simulink model "durumi2_model_Vt"  (R2022a)
settings: Solver=FixedStepAuto  StartTime=0.0  StopTime=10.0  FixedStep=0.01  RelTol=1e-3  EnableMultiTasking=on
values from neighbouring files (symbols this model uses):
  x0 = [100 0 0.646770657489 0 0 0 -0.000214853328121 0.00646761624384 -1.38957920864e-06 -7.89002982394e-16 -1.35365121342e-18 -499.999868019]    [durumi2_trim_100.mat]
undefined symbols (not defined in the file or in its folder): Alpha1, Alpha2, Beta1, Beta2, cbar, CD, CL, Cl_beta, CM, CM_alpha_dot, CN_beta, Ct1, CY_beta, dCD_da_In, dCD_da_Out, dCD_de, dCD_df, dCL_da_In, dCl_da_In, dCL_da_Out, dCl_da_Out, dCL_de, dCL_df, dCl_df, dCl_dr, dCl_p, dCL_q, dCl_r, dCM_da_In, dCM_da_Out, dCM_de, dCM_df, dCM_q, dCN_dr, dCN_p, dCN_r, dCY_dr, Del_Ail_In, Del_Ail_In_f, Del_Ail_Out, Del_Ail_Out_f, Del_Ele2, Del_Flap, Del_Rud, Dp, dxcg, dzcg, g, i_th, i_throttle, Inertia, Inertia_inv, J1, L_Ail_L_In, L_Ail_L_Out, L_Ail_R_In, L_Ail_R_Out, L_Flap_L, L_Flap_R, Mass ... (+7)
libraries: simulink_extras x3, matrix_library x2, aerospace x2
settings Model: Creator=김응태  LastModifiedBy=USer
settings DataIOCC: LimitDataPoints=on  SaveFormat=Array  SignalLoggingSaveFormat=ModelDataLogs  ReturnWorkspaceOutputs=off  SignalLoggingName=sigsOut
settings DebuggingCC: SaveWithParameterizedLinksMsg=none  MergeDetectMultiDrivingBlocksExec=none  SignalResolutionControl=TryResolveAllWithWarning  MultiTaskDSMMsg=warning  MultiTaskCondExecSysMsg=none  UnconnectedInputMsg=warning  UnconnectedOutputMsg=warning  UnconnectedLineMsg=warning
settings HardwareCC: ProdBitPerPointer=32  ProdBitPerSizeT=32  ProdBitPerPtrDiffT=32  ProdLargestAtomicFloat=None  ProdIntDivRoundTo=Undefined  ProdEndianess=Unspecified  ProdWordSize=32  ProdHWDeviceType=32-bit Generic  TargetUnknown=on
settings ModelReferenceCC: PropagateSignalLabelsOutOfModel=off
settings GRTTargetCC: CombineOutputUpdateFcns=off  GRTInterface=on
settings ConfigComp: CovMetricSettings=dw  CovSaveCumulativeToWorkspaceVar=on  CovSaveSingleToWorkspaceVar=on

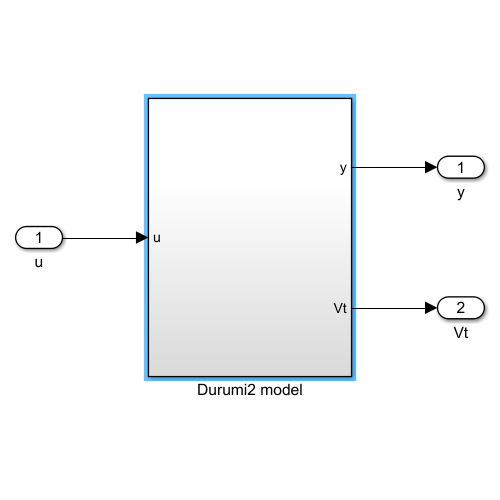
[thumbnail: Simulink's stored preview of the top-level diagram]
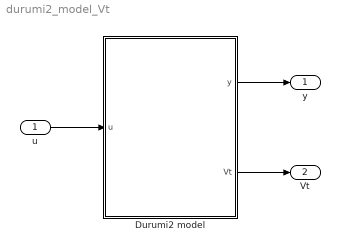
== system durumi2_model_Vt ==
  u : Inport
  Durumi2 model : Subsystem
  y : Outport
  Vt : Outport  Port=2
  wires:
  u/1 -> Durumi2 model/1(u)
  Durumi2 model/1(y) -> y/1
  Durumi2 model/2(Vt) -> Vt/1

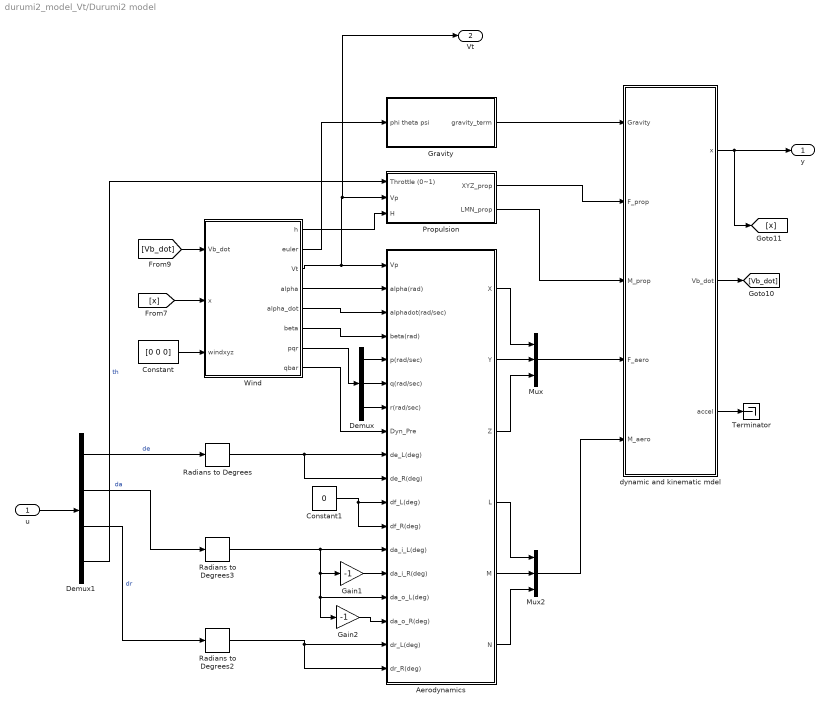
== system durumi2_model_Vt/Durumi2 model ==
  u : Inport
  "Aerodynamics " : Subsystem
  Constant : Constant  Value=[0 0 0]
  Constant1 : Constant  Value=0
  Demux : Demux  Outputs=3
      settings: DisplayOption=none
  Demux1 : Demux
  Gain1 : Gain  Gain=-1
  Gain2 : Gain  Gain=-1
  Gravity : Subsystem
  Mux : Mux  Inputs=3
  Mux2 : Mux  Inputs=3
  Propulsion : Subsystem
  Radians to Degrees : simulink_extras/Transformations/Radians to Degrees
  Radians to Degrees2 : simulink_extras/Transformations/Radians to Degrees
  Radians to Degrees3 : simulink_extras/Transformations/Radians to Degrees
  Terminator : Terminator
  Wind : Subsystem
  dynamic and kinematic mdel : Subsystem
  y : Outport
  Vt : Outport  Port=2
  wires:
  Wind/5(alpha_dot) -> "Aerodynamics "/3(alphadot(rad/sec))
  "Aerodynamics "/1(X) -> Mux/1
  Wind/8(qbar) -> "Aerodynamics "/8(Dyn_Pre)
  Wind/2(euler) -> Gravity/1(phi theta psi)
  Wind/6(beta) -> "Aerodynamics "/4(beta(rad))
  [x] -> Wind/2(x)
  [Vb_dot] -> Wind/1(Vb_dot)
  Propulsion/2(LMN_prop) -> dynamic and kinematic mdel/3(M_prop)
  Demux1/3 -> Radians to Degrees2/1  "dr"
  Propulsion/1(XYZ_prop) -> dynamic and kinematic mdel/2(F_prop)
  u/1 -> Demux1/1
  Radians to Degrees/1 -> "Aerodynamics "/10(de_R(deg)), "Aerodynamics "/9(de_L(deg))
  Constant1/1 -> "Aerodynamics "/12(df_R(deg)), "Aerodynamics "/11(df_L(deg))
  Demux1/1 -> Radians to Degrees/1  "de"
  dynamic and kinematic mdel/1(x) -> [x], y/1
  Constant/1 -> Wind/3(windxyz)
  Wind/7(pqr) -> Demux/1
  "Aerodynamics "/6(N) -> Mux2/3
  Demux/1 -> "Aerodynamics "/5(p(rad/sec))
  Wind/3(Vt) -> Vt/1, Propulsion/2(Vp), "Aerodynamics "/1(Vp)
  Demux1/2 -> Radians to Degrees3/1  "da"
  Gain2/1 -> "Aerodynamics "/16(da_o_R(deg))
  Demux/3 -> "Aerodynamics "/7(r(rad/sec))
  "Aerodynamics "/4(L) -> Mux2/1
  Mux/1 -> dynamic and kinematic mdel/4(F_aero)
  Gain1/1 -> "Aerodynamics "/14(da_i_R(deg))
  Wind/1(h) -> Propulsion/3(H)
  "Aerodynamics "/5(M) -> Mux2/2
  Gravity/1(gravity_term) -> dynamic and kinematic mdel/1(Gravity)
  dynamic and kinematic mdel/2(Vb_dot) -> [Vb_dot]
  Radians to Degrees3/1 -> "Aerodynamics "/13(da_i_L(deg)), Gain2/1, "Aerodynamics "/15(da_o_L(deg)), Gain1/1
  Demux/2 -> "Aerodynamics "/6(q(rad/sec))
  "Aerodynamics "/2(Y) -> Mux/2
  Demux1/4 -> Propulsion/1(Throttle (0~1))  "th"
  "Aerodynamics "/3(Z) -> Mux/3
  Wind/4(alpha) -> "Aerodynamics "/2(alpha(rad))
  Radians to Degrees2/1 -> "Aerodynamics "/17(dr_L(deg)), "Aerodynamics "/18(dr_R(deg))
  Mux2/1 -> dynamic and kinematic mdel/5(M_aero)
  dynamic and kinematic mdel/3(accel) -> Terminator/1

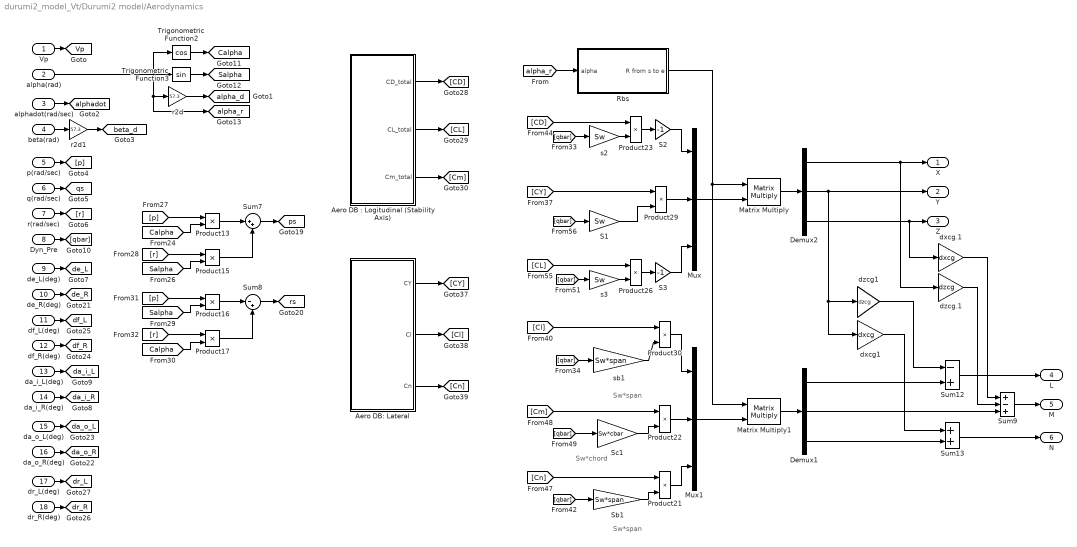
== system durumi2_model_Vt/Durumi2 model/Aerodynamics  ==
  note: Sw*span
  note: Sw*chord
  note: Sw*span
  Vp : Inport
  alpha(rad) : Inport  Port=2
  alphadot(rad/sec) : Inport  Port=3
  beta(rad) : Inport  Port=4
  p(rad/sec) : Inport  Port=5
  q(rad/sec) : Inport  Port=6
  r(rad/sec) : Inport  Port=7
  Dyn_Pre : Inport  Port=8
  de_L(deg) : Inport  Port=9
  de_R(deg) : Inport  Port=10
  df_L(deg) : Inport  Port=11
  df_R(deg) : Inport  Port=12
  da_i_L(deg) : Inport  Port=13
  da_i_R(deg) : Inport  Port=14
  da_o_L(deg) : Inport  Port=15
  da_o_R(deg) : Inport  Port=16
  dr_L(deg) : Inport  Port=17
  dr_R(deg) : Inport  Port=18
  "Aero DB : Logitudinal (Stability Axis)" : Subsystem
  Aero DB: Lateral : Subsystem
  Demux1 : Demux  Outputs=3
  Demux2 : Demux  Outputs=3
  Matrix Multiply : Product  Multiplication=Matrix(*)
  Matrix Multiply1 : Product  Multiplication=Matrix(*)
  Mux : Mux  Inputs=3
  Mux1 : Mux  Inputs=3
  Product{13,15..17,21..23,26,29..30} (10 alike) : Product  InputSameDT=on  SaturateOnIntegerOverflow=on  OutDataTypeStr=Inherit: Same as first input
  Rbs : Subsystem  AncestorBlock=|
      | aerolib6dofsys/DCM & Euler Angles (Euler)/phidot
      | thetadot
      | psidot
  S1 : Gain  Gain=Sw  SaturateOnIntegerOverflow=on  OutDataTypeStr=Inherit: Same as input  ParamDataTypeStr=Inherit: Same as input
  S2 : Gain  Gain=-1  SaturateOnIntegerOverflow=on  OutDataTypeStr=Inherit: Same as input  ParamDataTypeStr=Inherit: Same as input
  S3 : Gain  Gain=-1  SaturateOnIntegerOverflow=on  OutDataTypeStr=Inherit: Same as input  ParamDataTypeStr=Inherit: Same as input
  Sb1 : Gain  Gain=Sw*span  SaturateOnIntegerOverflow=on  OutDataTypeStr=Inherit: Same as input  ParamDataTypeStr=Inherit: Same as input
  Sc1 : Gain  Gain=Sw*cbar  SaturateOnIntegerOverflow=on  OutDataTypeStr=Inherit: Same as input  ParamDataTypeStr=Inherit: Same as input
  Sum12 : Sum  Inputs=-+  InputSameDT=on  SaturateOnIntegerOverflow=on  OutDataTypeStr=Inherit: Same as first input
  Sum13 : Sum  InputSameDT=on  SaturateOnIntegerOverflow=on  OutDataTypeStr=Inherit: Same as first input
  Sum7 : Sum  Inputs=|++  InputSameDT=on  SaturateOnIntegerOverflow=on  OutDataTypeStr=Inherit: Same as first input
  Sum8 : Sum  Inputs=|-+  InputSameDT=on  SaturateOnIntegerOverflow=on  OutDataTypeStr=Inherit: Same as first input
  Sum9 : Sum  Inputs=+-+  InputSameDT=on  SaturateOnIntegerOverflow=on  OutDataTypeStr=Inherit: Same as first input
  Trigonometric Function2 : Trigonometry  Operator=cos
  Trigonometric Function3 : Trigonometry
  dxcg.1 : Gain  Gain=dxcg  SaturateOnIntegerOverflow=on  OutDataTypeStr=Inherit: Same as input  ParamDataTypeStr=Inherit: Same as input
  dxcg1 : Gain  Gain=dxcg  SaturateOnIntegerOverflow=on  OutDataTypeStr=Inherit: Same as input  ParamDataTypeStr=Inherit: Same as input
  dzcg.1 : Gain  Gain=dzcg  SaturateOnIntegerOverflow=on  OutDataTypeStr=Inherit: Same as input  ParamDataTypeStr=Inherit: Same as input
  dzcg1 : Gain  Gain=dzcg  SaturateOnIntegerOverflow=on  OutDataTypeStr=Inherit: Same as input  ParamDataTypeStr=Inherit: Same as input
  r2d : Gain  Gain=57.3  SaturateOnIntegerOverflow=on  OutDataTypeStr=Inherit: Same as input  ParamDataTypeStr=Inherit: Same as input
  r2d1 : Gain  Gain=57.3  SaturateOnIntegerOverflow=on  OutDataTypeStr=Inherit: Same as input  ParamDataTypeStr=Inherit: Same as input
  s2 : Gain  Gain=Sw  SaturateOnIntegerOverflow=on  OutDataTypeStr=Inherit: Same as input  ParamDataTypeStr=Inherit: Same as input
  s3 : Gain  Gain=Sw  SaturateOnIntegerOverflow=on  OutDataTypeStr=Inherit: Same as input  ParamDataTypeStr=Inherit: Same as input
  sb1 : Gain  Gain=Sw*span  SaturateOnIntegerOverflow=on  OutDataTypeStr=Inherit: Same as input  ParamDataTypeStr=Inherit: Same as input
  X : Outport
  Y : Outport  Port=2
  Z : Outport  Port=3
  L : Outport  Port=4
  M : Outport  Port=5
  N : Outport  Port=6
  tag scope: Calpha=global, Salpha=global, Vp=global, alpha_d=global, alpha_r=global, alphadot=global, beta_d=global, da_i_L=global, da_i_R=global, da_o_L=global, da_o_R=global, de_L=global, de_R=global, df_L=global, df_R=global, dr_L=global, dr_R=global, ps=global, qs=global, rs=global
  wires:
  "Aero DB : Logitudinal (Stability Axis)"/3(Cm_total) -> [Cm]
  Aero DB: Lateral/3(Cn) -> [Cn]
  Aero DB: Lateral/2(Cl) -> [Cl]
  Aero DB: Lateral/1(CY) -> [CY]
  "Aero DB : Logitudinal (Stability Axis)"/2(CL_total) -> [CL]
  "Aero DB : Logitudinal (Stability Axis)"/1(CD_total) -> [CD]
  dr_R(deg)/1 -> [dr_R]
  dr_L(deg)/1 -> [dr_L]
  da_o_R(deg)/1 -> [da_o_R]
  da_o_L(deg)/1 -> [da_o_L]
  da_i_R(deg)/1 -> [da_i_R]
  da_i_L(deg)/1 -> [da_i_L]
  df_R(deg)/1 -> [df_R]
  df_L(deg)/1 -> [df_L]
  de_R(deg)/1 -> [de_R]
  Sum8/1 -> [rs]
  [r] -> Product17/1
  [p] -> Product16/1
  [Calpha] -> Product17/2
  [Salpha] -> Product16/2
  Product16/1 -> Sum8/1
  Product17/1 -> Sum8/2
  Sum7/1 -> [ps]
  [r] -> Product15/1
  [p] -> Product13/1
  [Salpha] -> Product15/2
  [Calpha] -> Product13/2
  Product13/1 -> Sum7/1
  Product15/1 -> Sum7/2
  Trigonometric Function3/1 -> [Salpha]
  Trigonometric Function2/1 -> [Calpha]
  r2d1/1 -> [beta_d]
  r2d/1 -> [alpha_d]
  Dyn_Pre/1 -> [qbar]
  alphadot(rad/sec)/1 -> [alphadot]
  beta(rad)/1 -> r2d1/1
  p(rad/sec)/1 -> [p]
  q(rad/sec)/1 -> [qs]
  r(rad/sec)/1 -> [r]
  de_L(deg)/1 -> [de_L]
  alpha(rad)/1 -> [alpha_r], r2d/1, Trigonometric Function2/1, Trigonometric Function3/1
  Vp/1 -> [Vp]
  Sb1/1 -> Product21/2
  [qbar] -> s2/1
  s3/1 -> Product26/2
  [qbar] -> S1/1
  Sc1/1 -> Product22/2
  [CD] -> Product23/1
  [CL] -> Product26/1
  s2/1 -> Product23/2
  [qbar] -> Sc1/1
  S1/1 -> Product29/2
  [qbar] -> sb1/1
  [Cl] -> Product30/1
  [CY] -> Product29/1
  [qbar] -> Sb1/1
  sb1/1 -> Product30/2
  [Cn] -> Product21/1
  [Cm] -> Product22/1
  [qbar] -> s3/1
  [alpha_r] -> Rbs/1(alpha)
  Rbs/1(R from s to e) -> Matrix Multiply/1, Matrix Multiply1/1
  Product29/1 -> Mux/2
  Product23/1 -> S2/1
  Product26/1 -> S3/1
  Product22/1 -> Mux1/2
  Product30/1 -> Mux1/1
  Product21/1 -> Mux1/3
  Mux1/1 -> Matrix Multiply1/2
  S2/1 -> Mux/1
  S3/1 -> Mux/3
  dzcg.1/1 -> Sum9/2
  dzcg1/1 -> Sum12/1
  Sum9/1 -> M/1
  Sum13/1 -> N/1
  Sum12/1 -> L/1
  Demux2/3 -> dxcg.1/1, Z/1
  Demux1/2 -> Sum9/3
  Demux1/1 -> Sum12/2
  Matrix Multiply/1 -> Demux2/1
  Matrix Multiply1/1 -> Demux1/1
  Demux2/2 -> dxcg1/1, dzcg1/1, Y/1
  dxcg.1/1 -> Sum9/1
  Demux2/1 -> X/1, dzcg.1/1
  dxcg1/1 -> Sum13/1
  Demux1/3 -> Sum13/2
  Mux/1 -> Matrix Multiply/2

== system durumi2_model_Vt/Durumi2 model/Gravity ==
  note: Gravaity
  phi theta psi : Inport
  . : Gain  Gain=g*Mass  SaturateOnIntegerOverflow=on  OutDataTypeStr=Inherit: Same as input  ParamDataTypeStr=Inherit: Same as input
  Mux : Mux  Inputs=3
  psidot2 : Fcn  Expr=cos(u[2])*cos(u[1])
  t : Fcn  Expr=-sin(u[2])
  tetadot : Fcn  Expr=cos(u[2])*sin(u[1])
  gravity_term : Outport  InitialOutput=0  VectorParamsAs1DForOutWhenUnconnected=off
  wires:
  t/1 -> Mux/1
  psidot2/1 -> Mux/3
  tetadot/1 -> Mux/2
  Mux/1 -> ./1
  phi theta psi/1 -> tetadot/1, t/1, psidot2/1
  ./1 -> gravity_term/1

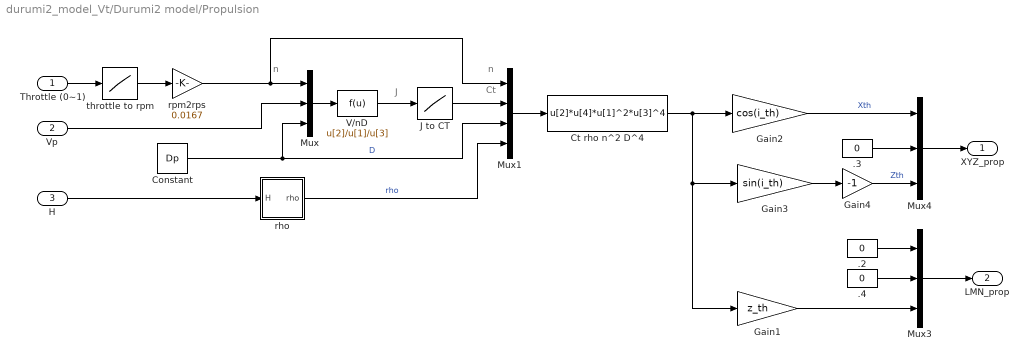
== system durumi2_model_Vt/Durumi2 model/Propulsion ==
  note: Ct
  note: n
  note: J
  note: n
  Throttle (0~1) : Inport
  Vp : Inport  Port=2
  H : Inport  Port=3
  .2 : Constant  Value=0  VectorParams1D=off
  .3 : Constant  Value=0  VectorParams1D=off
  .4 : Constant  Value=0  VectorParams1D=off
  Constant : Constant  Value=Dp
  Ct rho n^2 D^4 : Fcn  Expr=u[2]*u[4]*u[1]^2*u[3]^4
  Gain1 : Gain  Gain=z_th  SaturateOnIntegerOverflow=on  OutDataTypeStr=Inherit: Same as input  ParamDataTypeStr=Inherit: Same as input
  Gain2 : Gain  Gain=cos(i_th)  SaturateOnIntegerOverflow=on  OutDataTypeStr=Inherit: Same as input  ParamDataTypeStr=Inherit: Same as input
  Gain3 : Gain  Gain=sin(i_th)  SaturateOnIntegerOverflow=on  OutDataTypeStr=Inherit: Same as input  ParamDataTypeStr=Inherit: Same as input
  Gain4 : Gain  Gain=-1  SaturateOnIntegerOverflow=on  OutDataTypeStr=Inherit: Same as input  ParamDataTypeStr=Inherit: Same as input
  J to CT : Lookup  InputValues=J1  Table=Ct1
  Mux : Mux  Inputs=3
  Mux1 : Mux
  Mux3 : Mux  Inputs=3
  Mux4 : Mux  Inputs=3
  V/nD : Fcn  Expr=u[2]/u[1]/u[3]
  rho : Subsystem
  rpm2rps : Gain  Gain=0.0167  SaturateOnIntegerOverflow=on  OutDataTypeStr=Inherit: Same as input  ParamDataTypeStr=Inherit: Same as input
  throttle to rpm : Lookup  InputValues=i_throttle  Table=o_rpm
  XYZ_prop : Outport  VectorParamsAs1DForOutWhenUnconnected=off
  LMN_prop : Outport  Port=2  VectorParamsAs1DForOutWhenUnconnected=off
  wires:
  .3/1 -> Mux4/2
  Mux4/1 -> XYZ_prop/1
  Ct rho n^2 D^4/1 -> Gain2/1, Gain3/1, Gain1/1
  Gain1/1 -> Mux3/3
  Gain3/1 -> Gain4/1
  Mux3/1 -> LMN_prop/1
  .4/1 -> Mux3/2
  .2/1 -> Mux3/1
  Gain2/1 -> Mux4/1  "Xth"
  Gain4/1 -> Mux4/3  "Zth"
  rho/1(rho) -> Mux1/4  "rho"
  J to CT/1 -> Mux1/2
  Vp/1 -> Mux/2
  Mux/1 -> V/nD/1
  Mux1/1 -> Ct rho n^2 D^4/1
  V/nD/1 -> J to CT/1
  Constant/1 -> Mux1/3, Mux/3  "D"
  H/1 -> rho/1(H)
  Throttle (0~1)/1 -> throttle to rpm/1
  throttle to rpm/1 -> rpm2rps/1
  rpm2rps/1 -> Mux/1, Mux1/1

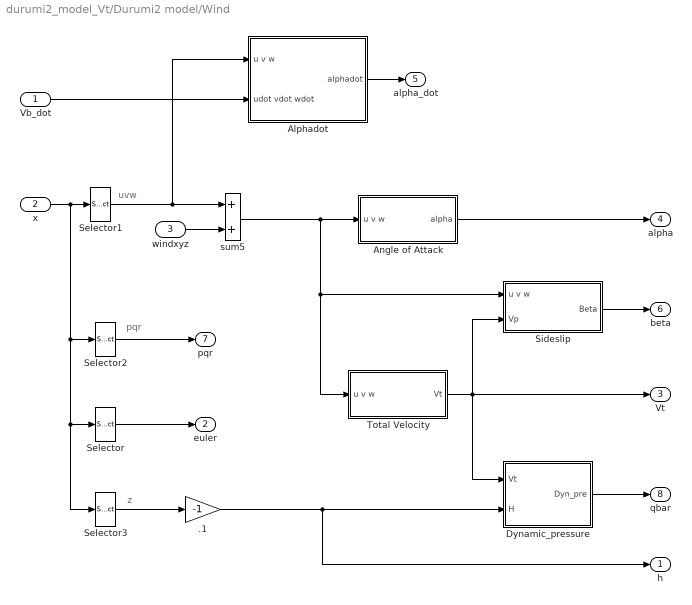
== system durumi2_model_Vt/Durumi2 model/Wind ==
  note: uvw
  note: pqr
  note: z
  Vb_dot : Inport
  x : Inport  Port=2
  windxyz : Inport  Port=3
  .1 : Gain  Gain=-1  OutDataTypeStr=Inherit: Same as input  ParamDataTypeStr=Inherit: Same as input
  Alphadot : Subsystem
  Angle of Attack : Subsystem
  Dynamic_pressure : Subsystem
  Selector : Selector  InputPortWidth=12  IndexOptions=Index vector (dialog)  Indices=[7 8 9]  OutputSizes=1
  Selector1 : Selector  InputPortWidth=12  IndexOptions=Index vector (dialog)  Indices=[1 2 3]  OutputSizes=1
  Selector2 : Selector  InputPortWidth=12  IndexOptions=Index vector (dialog)  Indices=[4 5 6]  OutputSizes=1
  Selector3 : Selector  InputPortWidth=12  IndexOptions=Index vector (dialog)  Indices=12  OutputSizes=1
  Sideslip : Subsystem
  Total Velocity : Subsystem
  sum5 : Sum  InputSameDT=on  SaturateOnIntegerOverflow=on  OutDataTypeStr=Inherit: Same as first input
  h : Outport  VectorParamsAs1DForOutWhenUnconnected=off
  euler : Outport  Port=2  VectorParamsAs1DForOutWhenUnconnected=off
  Vt : Outport  Port=3  VectorParamsAs1DForOutWhenUnconnected=off
  alpha : Outport  Port=4  VectorParamsAs1DForOutWhenUnconnected=off
  alpha_dot : Outport  Port=5  VectorParamsAs1DForOutWhenUnconnected=off
  beta : Outport  Port=6  VectorParamsAs1DForOutWhenUnconnected=off
  pqr : Outport  Port=7  VectorParamsAs1DForOutWhenUnconnected=off
  qbar : Outport  Port=8  VectorParamsAs1DForOutWhenUnconnected=off
  wires:
  x/1 -> Selector/1, Selector3/1, Selector2/1, Selector1/1
  Selector3/1 -> .1/1
  Angle of Attack/1(alpha) -> alpha/1
  Sideslip/1(Beta) -> beta/1
  windxyz/1 -> sum5/2
  Selector2/1 -> pqr/1
  sum5/1 -> Sideslip/1(u v w), Total Velocity/1(u v w), Angle of Attack/1(u v w)
  .1/1 -> Dynamic_pressure/2(H), h/1
  Total Velocity/1(Vt) -> Dynamic_pressure/1(Vt), Sideslip/2(Vp), Vt/1
  Dynamic_pressure/1(Dyn_pre) -> qbar/1
  Selector1/1 -> Alphadot/1(u v w), sum5/1
  Alphadot/1(alphadot) -> alpha_dot/1
  Vb_dot/1 -> Alphadot/2(udot vdot wdot)
  Selector/1 -> euler/1

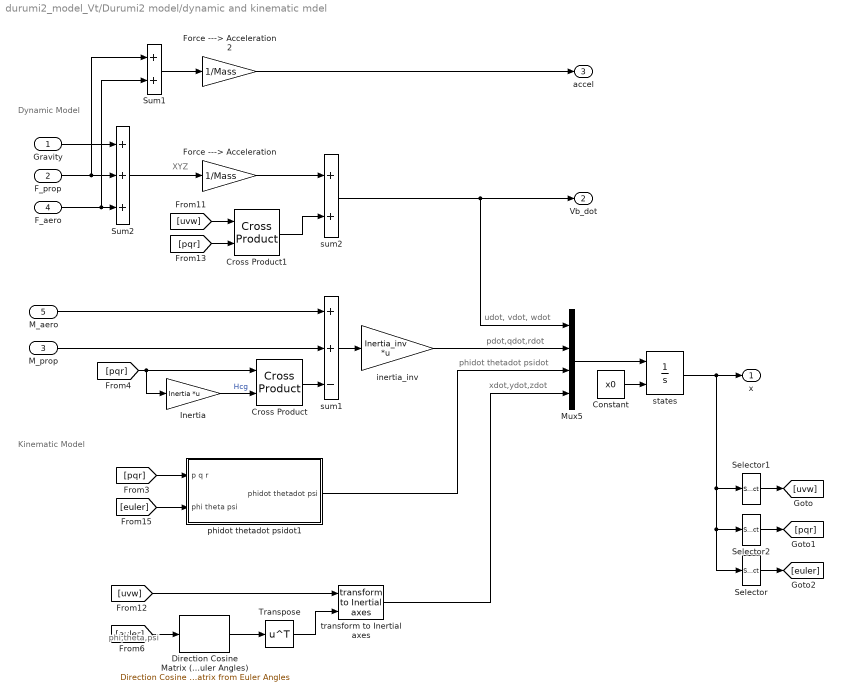
== system durumi2_model_Vt/Durumi2 model/dynamic and kinematic mdel ==
  note: Dynamic Model
  note: XYZ
  note: xdot,ydot,zdot
  note: phidot thetadot psidot
  note: pdot,qdot,rdot
  note: udot, vdot, wdot
  note: phi,theta,psi
  note: Kinematic Model
  Gravity : Inport
  F_prop : Inport  Port=2
  M_prop : Inport  Port=3
  F_aero : Inport  Port=4
  M_aero : Inport  Port=5
  Constant : Constant  Value=x0
  Cross Product : matrix_library/Cross Product
      settings: SourceProductBaseCode=SL
  Cross Product1 : matrix_library/Cross Product
      settings: SourceProductBaseCode=SL
  Direction Cosine Matrix (Euler Angles) : aerospace/Axes Transformations/Direction Cosine Matrix from Euler Angles
      settings: SourceProductBaseCode=SL
  Force ---> Acceleration : Gain  Gain=1/Mass  SaturateOnIntegerOverflow=on  OutDataTypeStr=Inherit: Same as input  ParamDataTypeStr=Inherit: Same as input
  Force ---> Acceleration2 : Gain  Gain=1/Mass  SaturateOnIntegerOverflow=on  OutDataTypeStr=Inherit: Same as input  ParamDataTypeStr=Inherit: Same as input
  Inertia : Gain  Gain=Inertia  Multiplication=Matrix(K*u)
  Mux5 : Mux
  Selector : Selector  InputPortWidth=12  IndexOptions=Index vector (dialog)  Indices=[7 8 9]  OutputSizes=1
  Selector1 : Selector  InputPortWidth=12  IndexOptions=Index vector (dialog)  Indices=[1 2 3]  OutputSizes=1
  Selector2 : Selector  InputPortWidth=12  IndexOptions=Index vector (dialog)  Indices=[4 5 6]  OutputSizes=1
  Sum1 : Sum  InputSameDT=on  SaturateOnIntegerOverflow=on  OutDataTypeStr=Inherit: Same as first input
  Sum2 : Sum  Inputs=+++  InputSameDT=on  SaturateOnIntegerOverflow=on  OutDataTypeStr=Inherit: Same as first input
  Transpose : Math  Operator=transpose  SignedPower=on
  inertia_inv : Gain  Gain=Inertia_inv  Multiplication=Matrix(K*u)
  phidot thetadot psidot1 : Subsystem  AncestorBlock=|
      | aerolib6dofsys/DCM & Euler Angles (Euler)/phidot
      | thetadot
      | psidot
  states : Integrator  InitialConditionSource=external  InitialCondition=x0
  sum1 : Sum  Inputs=++-  InputSameDT=on  SaturateOnIntegerOverflow=on  OutDataTypeStr=Inherit: Same as first input
  sum2 : Sum  InputSameDT=on  SaturateOnIntegerOverflow=on  OutDataTypeStr=Inherit: Same as first input
  "transform to Inertial axes " : aerospace/6DoF/Euler Angles/transform to Inertial axes   SystemSampleTime=-1  VariantActivationTime=update diagram  Latency=0  AutoFrameSizeCalculation=off
      settings: SourceProductBaseCode=SL
  x : Outport  VectorParamsAs1DForOutWhenUnconnected=off
  Vb_dot : Outport  Port=2  VectorParamsAs1DForOutWhenUnconnected=off
  accel : Outport  Port=3  VectorParamsAs1DForOutWhenUnconnected=off
  wires:
  Selector/1 -> [euler]
  Constant/1 -> states/2
  Selector1/1 -> [uvw]
  states/1 -> x/1, Selector2/1, Selector/1, Selector1/1
  Selector2/1 -> [pqr]
  [euler] -> Direction Cosine Matrix (Euler Angles)/1
  [pqr] -> phidot thetadot psidot1/1(p q r)
  "transform to Inertial axes "/1 -> Mux5/4
  [euler] -> phidot thetadot psidot1/2(phi theta psi)
  [pqr] -> Cross Product1/2
  [uvw] -> "transform to Inertial axes "/1
  [uvw] -> Cross Product1/1
  [pqr] -> Cross Product/1, Inertia/1
  Mux5/1 -> states/1
  inertia_inv/1 -> Mux5/2
  Transpose/1 -> "transform to Inertial axes "/2
  sum2/1 -> Vb_dot/1, Mux5/1
  Direction Cosine Matrix (Euler Angles)/1 -> Transpose/1
  phidot thetadot psidot1/1(phidot thetadot psi) -> Mux5/3
  Inertia/1 -> Cross Product/2  "Hcg"
  sum1/1 -> inertia_inv/1
  Cross Product1/1 -> sum2/2
  Force ---> Acceleration/1 -> sum2/1
  Sum2/1 -> Force ---> Acceleration/1
  F_prop/1 -> Sum1/1, Sum2/2
  F_aero/1 -> Sum1/2, Sum2/3
  M_aero/1 -> sum1/1
  Cross Product/1 -> sum1/3
  M_prop/1 -> sum1/2
  Sum1/1 -> Force ---> Acceleration2/1
  Gravity/1 -> Sum2/1
  Force ---> Acceleration2/1 -> accel/1

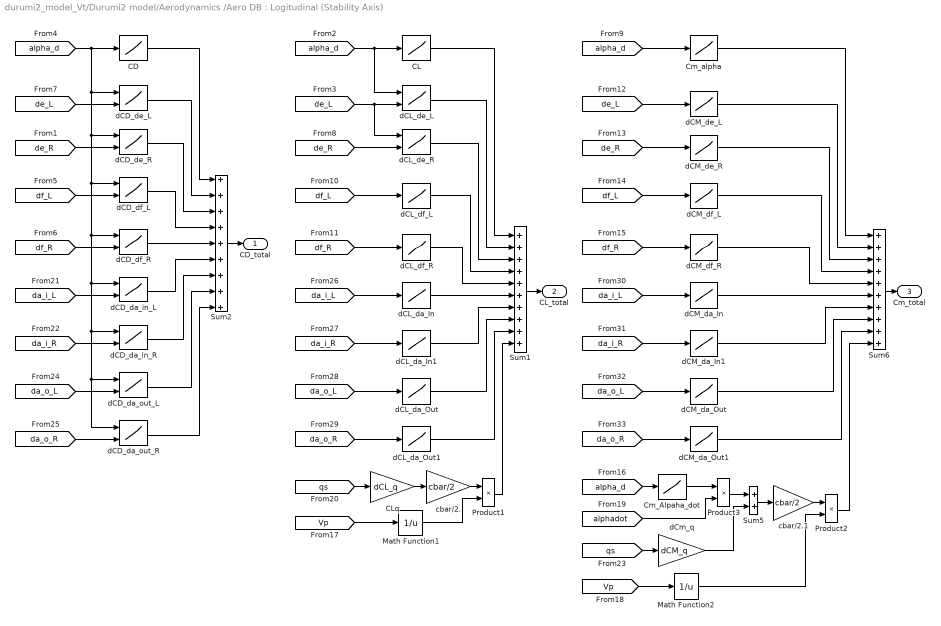
== system durumi2_model_Vt/Durumi2 model/Aerodynamics /Aero DB : Logitudinal (Stability Axis) ==
  CD : Lookup  InputValues=Alpha1  Table=CD
  CL : Lookup  InputValues=Alpha2  Table=CL
  CLq : Gain  Gain=dCL_q  SaturateOnIntegerOverflow=on  OutDataTypeStr=Inherit: Same as input  ParamDataTypeStr=Inherit: Same as input
  Cm_Alpaha_dot : Lookup  InputValues=Alpha2  Table=CM_alpha_dot
  Cm_alpha : Lookup  InputValues=Alpha2  Table=CM
  Math Function1 : Math  Operator=reciprocal  SignedPower=on
  Math Function2 : Math  Operator=reciprocal  SignedPower=on
  Product1 : Product  InputSameDT=on  SaturateOnIntegerOverflow=on  OutDataTypeStr=Inherit: Same as first input
  Product2 : Product  InputSameDT=on  SaturateOnIntegerOverflow=on  OutDataTypeStr=Inherit: Same as first input
  Product3 : Product  InputSameDT=on  SaturateOnIntegerOverflow=on  OutDataTypeStr=Inherit: Same as first input
  Sum1 : Sum  Inputs=++++++++++  InputSameDT=on  SaturateOnIntegerOverflow=on  OutDataTypeStr=Inherit: Same as first input
  Sum2 : Sum  Inputs=+++++++++  InputSameDT=on  SaturateOnIntegerOverflow=on  OutDataTypeStr=Inherit: Same as first input
  Sum5 : Sum  InputSameDT=on  SaturateOnIntegerOverflow=on  OutDataTypeStr=Inherit: Same as first input
  Sum6 : Sum  Inputs=++++++++++  InputSameDT=on  SaturateOnIntegerOverflow=on  OutDataTypeStr=Inherit: Same as first input
  cbar/2. : Gain  Gain=cbar/2  SaturateOnIntegerOverflow=on  OutDataTypeStr=Inherit: Same as input  ParamDataTypeStr=Inherit: Same as input
  cbar/2.1 : Gain  Gain=cbar/2  SaturateOnIntegerOverflow=on  OutDataTypeStr=Inherit: Same as input  ParamDataTypeStr=Inherit: Same as input
  dCD_da_in_L : Lookup2D  RowIndex=Alpha2  ColumnIndex=Del_Ail_In_f  Table=dCD_da_In  InputSameDT=off
  dCD_da_in_R : Lookup2D  RowIndex=Alpha2  ColumnIndex=Del_Ail_In_f  Table=dCD_da_In  InputSameDT=off
  dCD_da_out_L : Lookup2D  RowIndex=Alpha2  ColumnIndex=Del_Ail_Out_f  Table=dCD_da_Out  InputSameDT=off
  dCD_da_out_R : Lookup2D  RowIndex=Alpha2  ColumnIndex=Del_Ail_Out_f  Table=dCD_da_Out  InputSameDT=off
  dCD_de_L : Lookup2D  RowIndex=Alpha1  ColumnIndex=Del_Ele1  Table=dCD_de  InputSameDT=off
  dCD_de_R : Lookup2D  RowIndex=Alpha1  ColumnIndex=Del_Ele1  Table=dCD_de  InputSameDT=off
  dCD_df_L : Lookup2D  RowIndex=Alpha2  ColumnIndex=Del_Flap  Table=dCD_df  InputSameDT=off
  dCD_df_R : Lookup2D  RowIndex=Alpha2  ColumnIndex=Del_Flap  Table=dCD_df  InputSameDT=off
  dCL_da_In : Lookup  InputValues=Del_Ail_In_f  Table=dCL_da_In
  dCL_da_In1 : Lookup  InputValues=Del_Ail_In_f  Table=dCL_da_In
  dCL_da_Out : Lookup  InputValues=Del_Ail_Out_f  Table=dCL_da_Out
  dCL_da_Out1 : Lookup  InputValues=Del_Ail_Out_f  Table=dCL_da_Out
  dCL_de_L : Lookup2D  RowIndex=Alpha1  ColumnIndex=Del_Ele1  Table=dCL_de  InputSameDT=off
  dCL_de_R : Lookup2D  RowIndex=Alpha1  ColumnIndex=Del_Ele1  Table=dCL_de  InputSameDT=off
  dCL_df_L : Lookup  InputValues=Del_Flap  Table=dCL_df
  dCL_df_R : Lookup  InputValues=Del_Flap  Table=dCL_df
  dCM_da_In : Lookup  InputValues=Del_Ail_In_f  Table=dCM_da_In
  dCM_da_In1 : Lookup  InputValues=Del_Ail_In_f  Table=dCM_da_In
  dCM_da_Out : Lookup  InputValues=Del_Ail_Out_f  Table=dCM_da_Out
  dCM_da_Out1 : Lookup  InputValues=Del_Ail_Out_f  Table=dCM_da_Out
  dCM_de_L : Lookup  InputValues=Del_Ele2  Table=dCM_de
  dCM_de_R : Lookup  InputValues=Del_Ele2  Table=dCM_de
  dCM_df_L : Lookup  InputValues=Del_Flap  Table=dCM_df
  dCM_df_R : Lookup  InputValues=Del_Flap  Table=dCM_df
  dCm_q : Gain  Gain=dCM_q  SaturateOnIntegerOverflow=on  OutDataTypeStr=Inherit: Same as input  ParamDataTypeStr=Inherit: Same as input
  CD_total : Outport
  CL_total : Outport  Port=2
  Cm_total : Outport  Port=3
  wires:
  dCM_da_Out/1 -> Sum6/8
  dCM_da_In1/1 -> Sum6/7
  dCM_da_In/1 -> Sum6/6
  dCM_da_Out1/1 -> Sum6/9
  Product2/1 -> Sum6/10
  [da_o_R] -> dCM_da_Out1/1
  [da_o_L] -> dCM_da_Out/1
  [da_i_R] -> dCM_da_In1/1
  [da_i_L] -> dCM_da_In/1
  dCL_da_In1/1 -> Sum1/7
  dCL_da_Out/1 -> Sum1/8
  Product1/1 -> Sum1/10
  dCL_da_Out1/1 -> Sum1/9
  dCL_da_In/1 -> Sum1/6
  [da_o_R] -> dCL_da_Out1/1
  [da_o_L] -> dCL_da_Out/1
  [da_i_R] -> dCL_da_In1/1
  [da_i_L] -> dCL_da_In/1
  dCD_da_out_R/1 -> Sum2/9
  dCD_da_out_L/1 -> Sum2/8
  dCD_da_in_R/1 -> Sum2/7
  dCD_da_in_L/1 -> Sum2/6
  [da_o_R] -> dCD_da_out_R/2
  [da_o_L] -> dCD_da_out_L/2
  [da_i_R] -> dCD_da_in_R/2
  [da_i_L] -> dCD_da_in_L/2
  dCm_q/1 -> Sum5/2
  [alphadot] -> Product3/2
  Product3/1 -> Sum5/1
  Cm_Alpaha_dot/1 -> Product3/1
  Math Function1/1 -> Product1/2
  cbar/2./1 -> Product1/1
  CLq/1 -> cbar/2./1
  [Vp] -> Math Function1/1
  [qs] -> CLq/1
  dCM_de_L/1 -> Sum6/2
  Cm_alpha/1 -> Sum6/1
  dCM_df_R/1 -> Sum6/5
  dCM_de_R/1 -> Sum6/3
  dCM_df_L/1 -> Sum6/4
  Math Function2/1 -> Product2/2
  cbar/2.1/1 -> Product2/1
  Sum5/1 -> cbar/2.1/1
  [Vp] -> Math Function2/1
  [qs] -> dCm_q/1
  [alpha_d] -> Cm_Alpaha_dot/1
  [df_R] -> dCM_df_R/1
  [df_L] -> dCM_df_L/1
  [de_R] -> dCM_de_R/1
  [de_L] -> dCM_de_L/1
  [alpha_d] -> Cm_alpha/1
  Sum1/1 -> CL_total/1
  dCL_df_R/1 -> Sum1/5
  CL/1 -> Sum1/1
  dCL_df_L/1 -> Sum1/4
  dCL_de_L/1 -> Sum1/2
  dCL_de_R/1 -> Sum1/3
  [df_R] -> dCL_df_R/1
  [df_L] -> dCL_df_L/1
  [de_R] -> dCL_de_R/2
  [alpha_d] -> dCL_de_L/1, CL/1
  [df_R] -> dCD_df_R/2
  [df_L] -> dCD_df_L/2
  dCD_df_R/1 -> Sum2/5
  [de_R] -> dCD_de_R/2
  [de_L] -> dCD_de_L/2
  Sum6/1 -> Cm_total/1
  dCD_df_L/1 -> Sum2/4
  dCD_de_R/1 -> Sum2/3
  Sum2/1 -> CD_total/1
  dCD_de_L/1 -> Sum2/2
  CD/1 -> Sum2/1
  [alpha_d] -> dCD_da_out_R/1, dCD_da_out_L/1, dCD_da_in_R/1, dCD_da_in_L/1, dCD_df_R/1, dCD_df_L/1, dCD_de_R/1, dCD_de_L/1, CD/1
  [de_L] -> dCL_de_R/1, dCL_de_L/2

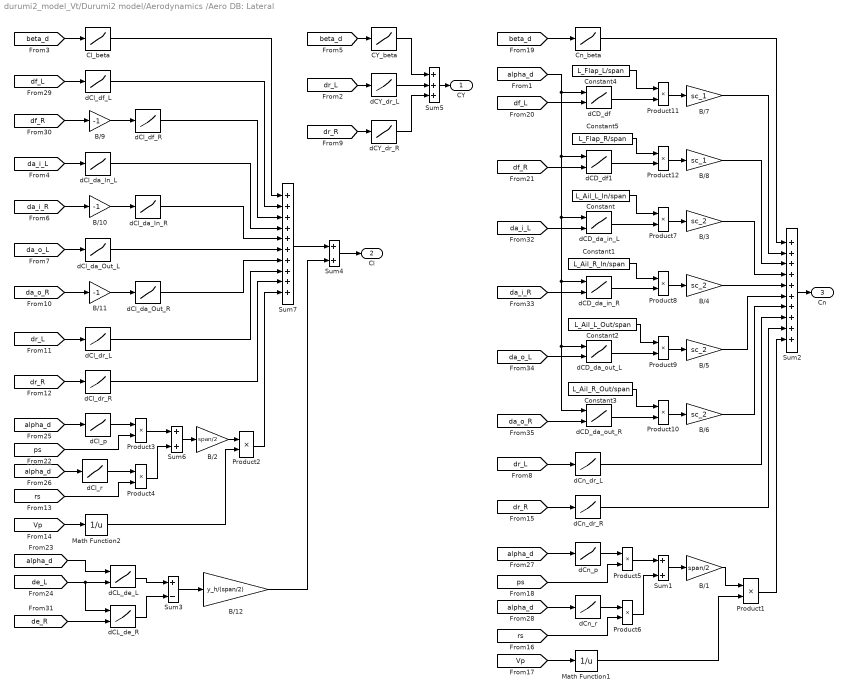
== system durumi2_model_Vt/Durumi2 model/Aerodynamics /Aero DB: Lateral ==
  B/1 : Gain  Gain=span/2  SaturateOnIntegerOverflow=on  OutDataTypeStr=Inherit: Same as input  ParamDataTypeStr=Inherit: Same as input
  B/10 : Gain  Gain=-1  SaturateOnIntegerOverflow=on  OutDataTypeStr=Inherit: Same as input  ParamDataTypeStr=Inherit: Same as input
  B/11 : Gain  Gain=-1  SaturateOnIntegerOverflow=on  OutDataTypeStr=Inherit: Same as input  ParamDataTypeStr=Inherit: Same as input
  B/12 : Gain  Gain=y_h/(span/2)  SaturateOnIntegerOverflow=on  OutDataTypeStr=Inherit: Same as input  ParamDataTypeStr=Inherit: Same as input
  B/2 : Gain  Gain=span/2  SaturateOnIntegerOverflow=on  OutDataTypeStr=Inherit: Same as input  ParamDataTypeStr=Inherit: Same as input
  B/{3..6} (4 alike) : Gain  Gain=sc_2  SaturateOnIntegerOverflow=on  OutDataTypeStr=Inherit: Same as input  ParamDataTypeStr=Inherit: Same as input
  B/7 : Gain  Gain=sc_1  SaturateOnIntegerOverflow=on  OutDataTypeStr=Inherit: Same as input  ParamDataTypeStr=Inherit: Same as input
  B/8 : Gain  Gain=sc_1  SaturateOnIntegerOverflow=on  OutDataTypeStr=Inherit: Same as input  ParamDataTypeStr=Inherit: Same as input
  B/9 : Gain  Gain=-1  SaturateOnIntegerOverflow=on  OutDataTypeStr=Inherit: Same as input  ParamDataTypeStr=Inherit: Same as input
  CY_beta : Lookup  InputValues=Beta1  Table=CY_beta
  Cl_beta : Lookup  InputValues=Beta2  Table=Cl_beta
  Cn_beta : Lookup  InputValues=Beta1  Table=CN_beta
  Constant : Constant  Value=L_Ail_L_In/span
  Constant1 : Constant  Value=L_Ail_R_In/span
  Constant2 : Constant  Value=L_Ail_L_Out/span
  Constant3 : Constant  Value=L_Ail_R_Out/span
  Constant4 : Constant  Value=L_Flap_L/span
  Constant5 : Constant  Value=L_Flap_R/span
  Math Function1 : Math  Operator=reciprocal  SignedPower=on
  Math Function2 : Math  Operator=reciprocal  SignedPower=on
  Product{1..12} (12 alike) : Product  InputSameDT=on  SaturateOnIntegerOverflow=on  OutDataTypeStr=Inherit: Same as first input
  Sum1 : Sum  InputSameDT=on  SaturateOnIntegerOverflow=on  OutDataTypeStr=Inherit: Same as first input
  Sum2 : Sum  Inputs=++++++++++  InputSameDT=on  SaturateOnIntegerOverflow=on  OutDataTypeStr=Inherit: Same as first input
  Sum3 : Sum  Inputs=+-  InputSameDT=on  SaturateOnIntegerOverflow=on  OutDataTypeStr=Inherit: Same as first input
  Sum4 : Sum  InputSameDT=on  SaturateOnIntegerOverflow=on  OutDataTypeStr=Inherit: Same as first input
  Sum5 : Sum  Inputs=+++  InputSameDT=on  SaturateOnIntegerOverflow=on  OutDataTypeStr=Inherit: Same as first input
  Sum6 : Sum  InputSameDT=on  SaturateOnIntegerOverflow=on  OutDataTypeStr=Inherit: Same as first input
  Sum7 : Sum  Inputs=++++++++++  InputSameDT=on  SaturateOnIntegerOverflow=on  OutDataTypeStr=Inherit: Same as first input
  dCD_da_in_L : Lookup2D  RowIndex=Alpha2  ColumnIndex=Del_Ail_In_f  Table=dCD_da_In  InputSameDT=off
  dCD_da_in_R : Lookup2D  RowIndex=Alpha2  ColumnIndex=Del_Ail_In_f  Table=dCD_da_In  InputSameDT=off
  dCD_da_out_L : Lookup2D  RowIndex=Alpha2  ColumnIndex=Del_Ail_Out_f  Table=dCD_da_Out  InputSameDT=off
  dCD_da_out_R : Lookup2D  RowIndex=Alpha2  ColumnIndex=Del_Ail_Out_f  Table=dCD_da_Out  InputSameDT=off
  dCD_df : Lookup2D  RowIndex=Alpha2  ColumnIndex=Del_Flap  Table=dCD_df  InputSameDT=off
  dCD_df1 : Lookup2D  RowIndex=Alpha2  ColumnIndex=Del_Flap  Table=dCD_df  InputSameDT=off
  dCL_de_L : Lookup2D  RowIndex=Alpha1  ColumnIndex=Del_Ele1  Table=dCL_de  InputSameDT=off
  dCL_de_R : Lookup2D  RowIndex=Alpha1  ColumnIndex=Del_Ele1  Table=dCL_de  InputSameDT=off
  dCY_dr_L : Lookup  InputValues=Del_Rud  Table=dCY_dr
  dCY_dr_R : Lookup  InputValues=Del_Rud  Table=dCY_dr
  dCl_da_In_L : Lookup  InputValues=Del_Ail_In  Table=dCl_da_In
  dCl_da_In_R : Lookup  InputValues=Del_Ail_In  Table=dCl_da_In
  dCl_da_Out_L : Lookup  InputValues=Del_Ail_Out  Table=dCl_da_Out
  dCl_da_Out_R : Lookup  InputValues=Del_Ail_Out  Table=dCl_da_Out
  dCl_df_L : Lookup  InputValues=Del_Flap  Table=dCl_df
  dCl_df_R : Lookup  InputValues=Del_Flap  Table=dCl_df
  dCl_dr_L : Lookup  InputValues=Del_Rud  Table=dCl_dr
  dCl_dr_R : Lookup  InputValues=Del_Rud  Table=dCl_dr
  dCl_p : Lookup  InputValues=Alpha2  Table=dCl_p
  dCl_r : Lookup  InputValues=Alpha2  Table=dCl_r
  dCn_dr_L : Lookup  InputValues=Del_Rud  Table=dCN_dr
  dCn_dr_R : Lookup  InputValues=Del_Rud  Table=dCN_dr
  dCn_p : Lookup  InputValues=Alpha2  Table=dCN_p
  dCn_r : Lookup  InputValues=Alpha2  Table=dCN_r
  CY : Outport
  Cl : Outport  Port=2
  Cn : Outport  Port=3
  wires:
  B/12/1 -> Sum4/2
  Sum3/1 -> B/12/1
  Sum4/1 -> Cl/1
  Sum7/1 -> Sum4/1
  dCL_de_R/1 -> Sum3/2
  dCL_de_L/1 -> Sum3/1
  [de_R] -> dCL_de_R/2
  [alpha_d] -> dCL_de_L/1
  [de_L] -> dCL_de_R/1, dCL_de_L/2
  B/11/1 -> dCl_da_Out_R/1
  B/10/1 -> dCl_da_In_R/1
  B/9/1 -> dCl_df_R/1
  Product1/1 -> Sum2/10
  dCn_dr_R/1 -> Sum2/9
  dCn_dr_L/1 -> Sum2/8
  B/6/1 -> Sum2/7
  B/5/1 -> Sum2/6
  B/4/1 -> Sum2/5
  B/3/1 -> Sum2/4
  B/8/1 -> Sum2/3
  B/7/1 -> Sum2/2
  Product12/1 -> B/8/1
  Product11/1 -> B/7/1
  Constant5/1 -> Product12/1
  dCD_df1/1 -> Product12/2
  Constant4/1 -> Product11/1
  dCD_df/1 -> Product11/2
  [df_R] -> dCD_df1/2
  [df_L] -> dCD_df/2
  [alpha_d] -> dCD_da_out_R/1, dCD_da_out_L/1, dCD_da_in_R/1, dCD_da_in_L/1, dCD_df1/1, dCD_df/1
  Product10/1 -> B/6/1
  Product9/1 -> B/5/1
  Product8/1 -> B/4/1
  Product7/1 -> B/3/1
  [alpha_d] -> dCl_r/1
  B/2/1 -> Product2/1
  Constant3/1 -> Product10/1
  dCD_da_out_R/1 -> Product10/2
  dCD_da_out_L/1 -> Product9/2
  Constant2/1 -> Product9/1
  Constant1/1 -> Product8/1
  dCD_da_in_R/1 -> Product8/2
  Constant/1 -> Product7/1
  dCD_da_in_L/1 -> Product7/2
  [da_o_R] -> dCD_da_out_R/2
  [da_o_L] -> dCD_da_out_L/2
  [da_i_R] -> dCD_da_in_R/2
  [da_i_L] -> dCD_da_in_L/2
  dCl_da_Out_R/1 -> Sum7/7
  dCl_dr_L/1 -> Sum7/8
  dCl_dr_R/1 -> Sum7/9
  Product2/1 -> Sum7/10
  dCl_da_In_R/1 -> Sum7/5
  dCl_da_In_L/1 -> Sum7/4
  dCl_df_R/1 -> Sum7/3
  dCl_df_L/1 -> Sum7/2
  dCl_da_Out_L/1 -> Sum7/6
  [df_R] -> B/9/1
  [df_L] -> dCl_df_L/1
  [Vp] -> Math Function1/1
  Product6/1 -> Sum1/2
  [ps] -> Product5/2
  Product5/1 -> Sum1/1
  [rs] -> Product6/2
  dCn_r/1 -> Product6/1
  [alpha_d] -> dCn_r/1
  dCn_p/1 -> Product5/1
  [alpha_d] -> dCn_p/1
  [Vp] -> Math Function2/1
  Product4/1 -> Sum6/2
  [rs] -> Product4/2
  dCl_r/1 -> Product4/1
  [ps] -> Product3/2
  dCl_p/1 -> Product3/1
  [alpha_d] -> dCl_p/1
  Product3/1 -> Sum6/1
  Cn_beta/1 -> Sum2/1
  Sum2/1 -> Cn/1
  Math Function1/1 -> Product1/2
  B/1/1 -> Product1/1
  Sum1/1 -> B/1/1
  [dr_R] -> dCn_dr_R/1
  [dr_L] -> dCn_dr_L/1
  [beta_d] -> Cn_beta/1
  Cl_beta/1 -> Sum7/1
  Math Function2/1 -> Product2/2
  Sum6/1 -> B/2/1
  [dr_R] -> dCl_dr_R/1
  [dr_L] -> dCl_dr_L/1
  [da_o_R] -> B/11/1
  [da_o_L] -> dCl_da_Out_L/1
  [da_i_R] -> B/10/1
  [da_i_L] -> dCl_da_In_L/1
  [beta_d] -> Cl_beta/1
  dCY_dr_R/1 -> Sum5/3
  CY_beta/1 -> Sum5/1
  [dr_R] -> dCY_dr_R/1
  [dr_L] -> dCY_dr_L/1
  dCY_dr_L/1 -> Sum5/2
  [beta_d] -> CY_beta/1
  Sum5/1 -> CY/1

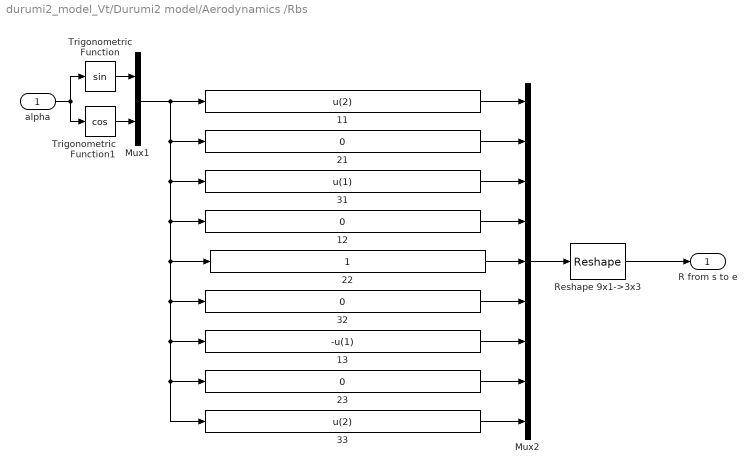
== system durumi2_model_Vt/Durumi2 model/Aerodynamics /Rbs ==
  alpha : Inport
  11 : Fcn  Expr=u(2)
  {12,21,23,32} (4 alike) : Fcn  Expr=0
  13 : Fcn  Expr=-u(1)
  22 : Fcn  Expr=1
  31 : Fcn  Expr=u(1)
  33 : Fcn  Expr=u(2)
  Mux1 : Mux  Inputs=2
  Mux2 : Mux  Inputs=9
  Reshape 9x1->3x3 : Reshape  OutputDimensionality=Customize  OutputDimensions=[3,3]
  Trigonometric Function : Trigonometry
  Trigonometric Function1 : Trigonometry  Operator=cos
  R from s to e : Outport  InitialOutput=0  VectorParamsAs1DForOutWhenUnconnected=off
  wires:
  Trigonometric Function1/1 -> Mux1/2
  Trigonometric Function/1 -> Mux1/1
  Reshape 9x1->3x3/1 -> R from s to e/1
  alpha/1 -> Trigonometric Function1/1, Trigonometric Function/1
  11/1 -> Mux2/1
  Mux2/1 -> Reshape 9x1->3x3/1
  21/1 -> Mux2/2
  22/1 -> Mux2/5
  Mux1/1 -> 23/1, 33/1, 13/1, 32/1, 22/1, 12/1, 31/1, 21/1, 11/1
  13/1 -> Mux2/7
  32/1 -> Mux2/6
  12/1 -> Mux2/4
  33/1 -> Mux2/9
  23/1 -> Mux2/8
  31/1 -> Mux2/3

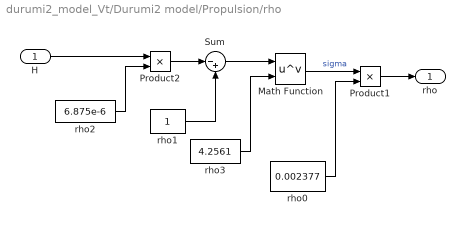
== system durumi2_model_Vt/Durumi2 model/Propulsion/rho ==
  H : Inport
  Math Function : Math  Operator=pow  SignedPower=on
  Product1 : Product  InputSameDT=on  SaturateOnIntegerOverflow=on  OutDataTypeStr=Inherit: Same as first input
  Product2 : Product  InputSameDT=on  SaturateOnIntegerOverflow=on  OutDataTypeStr=Inherit: Same as first input
  Sum : Sum  Inputs=|-+  SaturateOnIntegerOverflow=on
  rho0 : Constant  Value=0.002377
  rho1 : Constant
  rho2 : Constant  Value=6.875e-6
  rho3 : Constant  Value=4.2561
  rho : Outport
  wires:
  H/1 -> Product2/1
  rho0/1 -> Product1/2
  rho1/1 -> Sum/2
  Product2/1 -> Sum/1
  Sum/1 -> Math Function/1
  rho3/1 -> Math Function/2
  Math Function/1 -> Product1/1  "sigma"
  Product1/1 -> rho/1
  rho2/1 -> Product2/2

== system durumi2_model_Vt/Durumi2 model/Wind/Alphadot ==
  u v w : Inport
  udot vdot wdot : Inport  Port=2
  Mux : Mux  Inputs=2
  dalpha : Fcn  Expr=(u[1]*u[6]-u[4]*u[3])/(u[1]^2+u[3]^2)
  alphadot : Outport  InitialOutput=0  VectorParamsAs1DForOutWhenUnconnected=off
  wires:
  dalpha/1 -> alphadot/1
  Mux/1 -> dalpha/1
  u v w/1 -> Mux/1
  udot vdot wdot/1 -> Mux/2

== system durumi2_model_Vt/Durumi2 model/Wind/Angle of Attack ==
  u v w : Inport
  Vel : Fcn  Expr=atan(u[3]/u[1])
  alpha : Outport  InitialOutput=0  VectorParamsAs1DForOutWhenUnconnected=off
  wires:
  u v w/1 -> Vel/1
  Vel/1 -> alpha/1

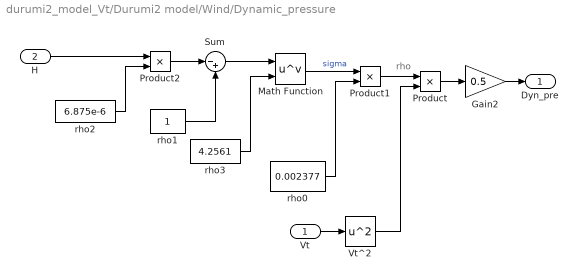
== system durumi2_model_Vt/Durumi2 model/Wind/Dynamic_pressure ==
  note: rho
  Vt : Inport
  H : Inport  Port=2
  Gain2 : Gain  Gain=0.5  SaturateOnIntegerOverflow=on  OutDataTypeStr=Inherit: Same as input  ParamDataTypeStr=Inherit: Same as input
  Math Function : Math  Operator=pow  SignedPower=on
  Product : Product  InputSameDT=on  SaturateOnIntegerOverflow=on  OutDataTypeStr=Inherit: Same as first input
  Product1 : Product  InputSameDT=on  SaturateOnIntegerOverflow=on  OutDataTypeStr=Inherit: Same as first input
  Product2 : Product  InputSameDT=on  SaturateOnIntegerOverflow=on  OutDataTypeStr=Inherit: Same as first input
  Sum : Sum  Inputs=|-+  SaturateOnIntegerOverflow=on
  Vt^2 : Math  Operator=square  SignedPower=on
  rho0 : Constant  Value=0.002377
  rho1 : Constant
  rho2 : Constant  Value=6.875e-6
  rho3 : Constant  Value=4.2561
  Dyn_pre : Outport
  wires:
  rho2/1 -> Product2/2
  Gain2/1 -> Dyn_pre/1
  Math Function/1 -> Product1/1  "sigma"
  Product1/1 -> Product/1
  rho3/1 -> Math Function/2
  Sum/1 -> Math Function/1
  Product2/1 -> Sum/1
  rho1/1 -> Sum/2
  rho0/1 -> Product1/2
  Product/1 -> Gain2/1
  Vt^2/1 -> Product/2
  Vt/1 -> Vt^2/1
  H/1 -> Product2/1

== system durumi2_model_Vt/Durumi2 model/Wind/Sideslip ==
  u v w : Inport
  Vp : Inport  Port=2
  Mux : Mux  Inputs=2
  beta : Fcn  Expr=asin(u[2]/u[4])
  Beta : Outport  InitialOutput=0  VectorParamsAs1DForOutWhenUnconnected=off
  wires:
  Mux/1 -> beta/1
  beta/1 -> Beta/1
  Vp/1 -> Mux/2
  u v w/1 -> Mux/1

== system durumi2_model_Vt/Durumi2 model/Wind/Total Velocity ==
  u v w : Inport
  Vel : Fcn  Expr=sqrt(u[1]^2+u[2]^2+u[3]^2)
  Vt : Outport  InitialOutput=0  VectorParamsAs1DForOutWhenUnconnected=off
  wires:
  u v w/1 -> Vel/1
  Vel/1 -> Vt/1

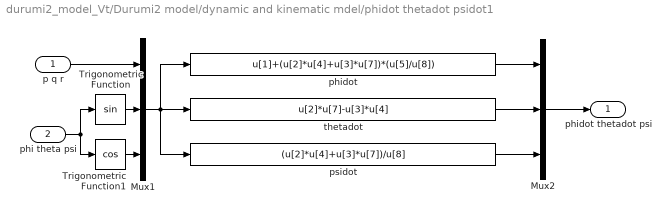
== system durumi2_model_Vt/Durumi2 model/dynamic and kinematic mdel/phidot thetadot psidot1 ==
  p q r : Inport
  phi theta psi : Inport  Port=2
  Mux1 : Mux  Inputs=[3 3 3]
  Mux2 : Mux  Inputs=3
  Trigonometric Function : Trigonometry
  Trigonometric Function1 : Trigonometry  Operator=cos
  phidot : Fcn  Expr=u[1]+(u[2]*u[4]+u[3]*u[7])*(u[5]/u[8])
  psidot : Fcn  Expr=(u[2]*u[4]+u[3]*u[7])/u[8]
  thetadot : Fcn  Expr=u[2]*u[7]-u[3]*u[4]
  phidot thetadot psi : Outport  InitialOutput=0  VectorParamsAs1DForOutWhenUnconnected=off
  wires:
  Trigonometric Function1/1 -> Mux1/3
  Trigonometric Function/1 -> Mux1/2
  Mux2/1 -> phidot thetadot psi/1
  phidot/1 -> Mux2/1
  thetadot/1 -> Mux2/2
  psidot/1 -> Mux2/3
  phi theta psi/1 -> Trigonometric Function1/1, Trigonometric Function/1
  p q r/1 -> Mux1/1
  Mux1/1 -> thetadot/1, phidot/1, psidot/1
